simulink model "Lab3_OpenLoop"  (R2016a)
settings: Solver=VariableStepAuto  StartTime=0.0  StopTime=10.0  RelTol=1e-3
libraries: simulink x1
settings Model: Creator=jordan  LastModifiedBy=jordan

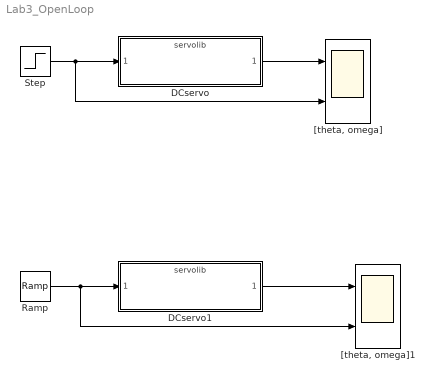
== system Lab3_OpenLoop ==
  DCservo : ModelReference  ModelNameDialog=servolib.slx  SimulationMode=Normal  ModelReferenceVersion=1.56
  DCservo1 : ModelReference  ModelNameDialog=servolib.slx  SimulationMode=Normal  ModelReferenceVersion=1.56
  Ramp : simulink/Sources/Ramp  slope=1  start=0  X0=0
  Step : Step  SampleTime=0
  "[theta, omega]" : Scope  NumInputPorts=2
  "[theta, omega]1" : Scope  NumInputPorts=2
  wires:
  DCservo/1 -> "[theta, omega]"/1
  Step/1 -> "[theta, omega]"/2, DCservo/1
  DCservo1/1 -> "[theta, omega]1"/1
  Ramp/1 -> "[theta, omega]1"/2, DCservo1/1
